simulink model "UAV_SIL"  (R2016b)
settings: Solver=VariableStepAuto  StartTime=0.0  StopTime=10.0  RelTol=1e-3
values from neighbouring files (symbols this model uses):
  MPCSampleTime = 0.02    [matlab.mat]    (also in setup.m)
  TrimCondition =     [matlab.mat]
libraries: Controller_Wrapper x1, Actuator_Lib x1, AircraftModel x1
settings Model: Creator=UAVLAB  LastModifiedBy=UAVLAB

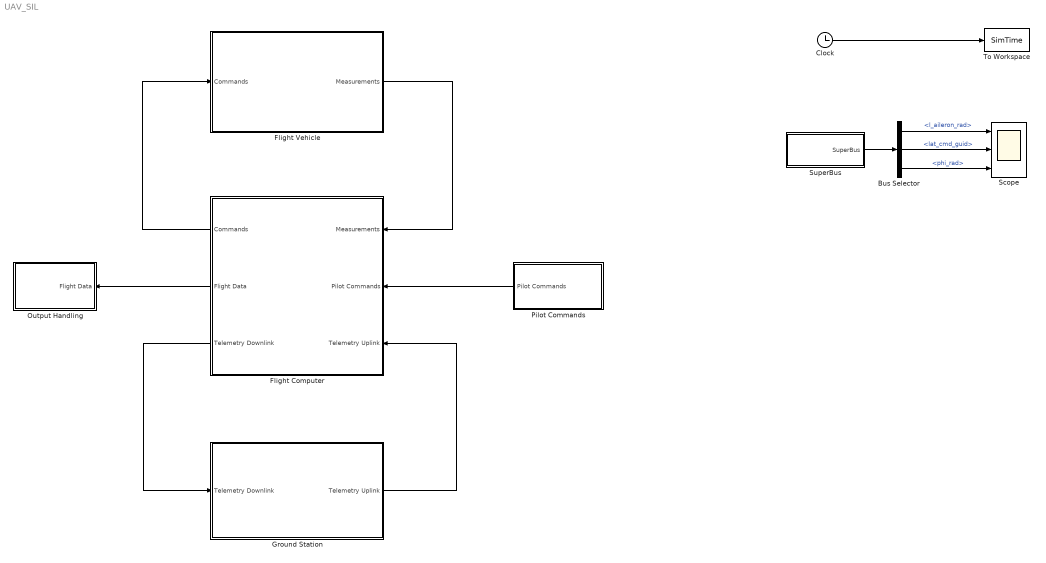
== system UAV_SIL ==
  Bus Selector : BusSelector  OutputSignals=Actuator States.CtrlSurf.l_aileron_rad,References.lat_cmd_guid,Aircraft States.RigidStates.Euler.phi_rad
  Clock : Clock
  Flight Computer : Subsystem
  Flight Vehicle : Subsystem
  Ground Station : Subsystem
  Output Handling : Subsystem
  Pilot Commands : Subsystem
  Scope : Scope  NumInputPorts=3
  SuperBus : Subsystem
  To Workspace : ToWorkspace  VariableName=SimTime  SampleTime=-1
  wires:
  Clock/1 -> To Workspace/1
  SuperBus/1(SuperBus) -> Bus Selector/1
  Flight Vehicle/1(Measurements) -> Flight Computer/1(Measurements)
  Pilot Commands/1(Pilot Commands) -> Flight Computer/2(Pilot Commands)
  Ground Station/1(Telemetry Uplink) -> Flight Computer/3(Telemetry Uplink)
  Flight Computer/1(Commands) -> Flight Vehicle/1(Commands)
  Flight Computer/3(Telemetry Downlink) -> Ground Station/1(Telemetry Downlink)
  Flight Computer/2(Flight Data) -> Output Handling/1(Flight Data)
  Bus Selector/1 -> Scope/1  "<l_aileron_rad>"
  Bus Selector/2 -> Scope/2  "<lat_cmd_guid>"
  Bus Selector/3 -> Scope/3  "<phi_rad>"

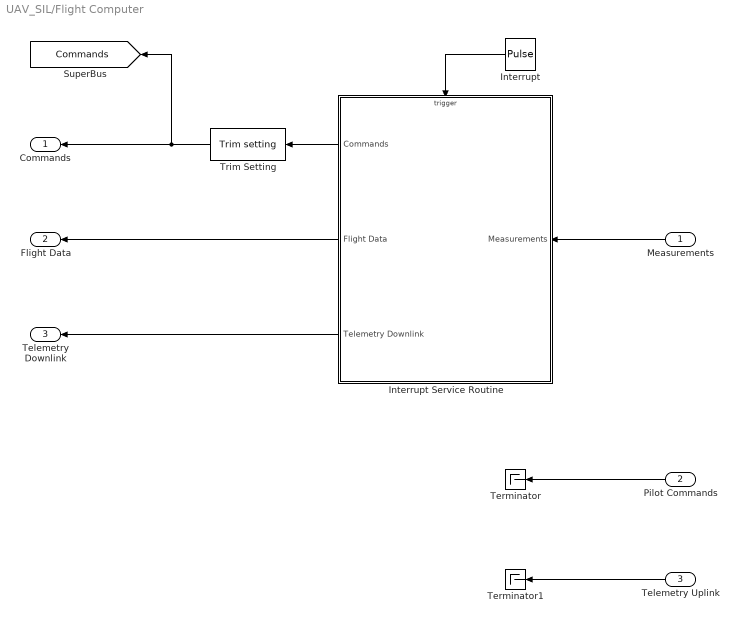
== system UAV_SIL/Flight Computer ==
  Measurements : Inport  OutDataTypeStr=Bus: Sensors
  Pilot Commands : Inport  Port=2  OutDataTypeStr=Bus: PilotCommands
  Telemetry Uplink : Inport  Port=3
  Interrupt : DiscretePulseGenerator  PulseType=Time based  Period=MPCSampleTime  PulseWidth=5
  Interrupt Service Routine : Subsystem  TreatAsAtomicUnit=on
  Terminator : Terminator
  Terminator1 : Terminator
  "Trim Setting " : Actuator_Lib/Trim setting 
  Commands : Outport  OutDataTypeStr=Bus: Commands
  Flight Data : Outport  Port=2
  Telemetry Downlink : Outport  Port=3
  tag scope: Commands=global
  wires:
  Interrupt/1 -> Interrupt Service Routine/Trigger
  Measurements/1 -> Interrupt Service Routine/1(Measurements)
  Interrupt Service Routine/1(Commands) -> "Trim Setting "/1
  "Trim Setting "/1 -> [Commands], Commands/1
  Pilot Commands/1 -> Terminator/1
  Interrupt Service Routine/2(Flight Data) -> Flight Data/1
  Interrupt Service Routine/3(Telemetry Downlink) -> Telemetry Downlink/1
  Telemetry Uplink/1 -> Terminator1/1

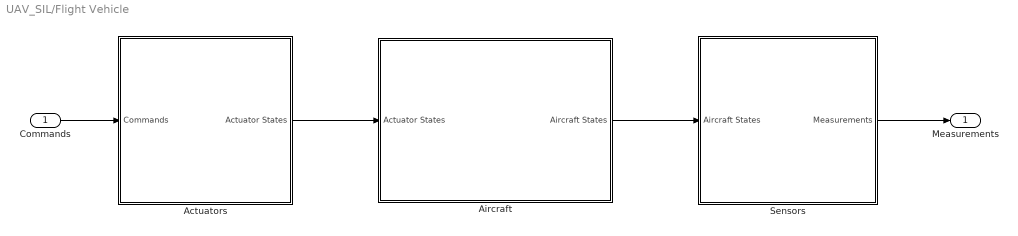
== system UAV_SIL/Flight Vehicle ==
  Commands : Inport  OutDataTypeStr=Bus: Commands
  Actuators : Subsystem
  Aircraft : Subsystem
  Sensors : Subsystem
  Measurements : Outport  OutDataTypeStr=Bus: Sensors  LockScale=on
  wires:
  Sensors/1(Measurements) -> Measurements/1
  Commands/1 -> Actuators/1(Commands)
  Actuators/1(Actuator States) -> Aircraft/1(Actuator States)
  Aircraft/1(Aircraft States) -> Sensors/1(Aircraft States)

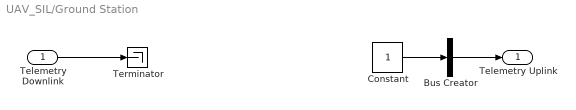
== system UAV_SIL/Ground Station ==
  Telemetry Downlink : Inport
  Bus Creator : BusCreator  Inputs=1
  Constant : Constant
  Terminator : Terminator
  Telemetry Uplink : Outport
  wires:
  Telemetry Downlink/1 -> Terminator/1
  Constant/1 -> Bus Creator/1
  Bus Creator/1 -> Telemetry Uplink/1

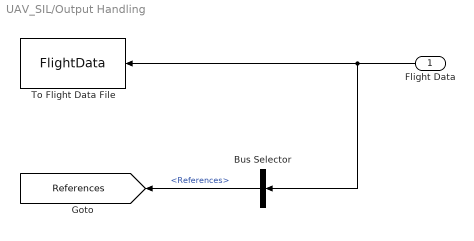
== system UAV_SIL/Output Handling ==
  Flight Data : Inport
  Bus Selector : BusSelector  OutputSignals=References
  To Flight Data File : ToWorkspace  VariableName=FlightData  SaveFormat=Structure With Time  SampleTime=-1
  tag scope: References=global
  wires:
  Flight Data/1 -> Bus Selector/1, To Flight Data File/1
  Bus Selector/1 -> [References]  "<References>"

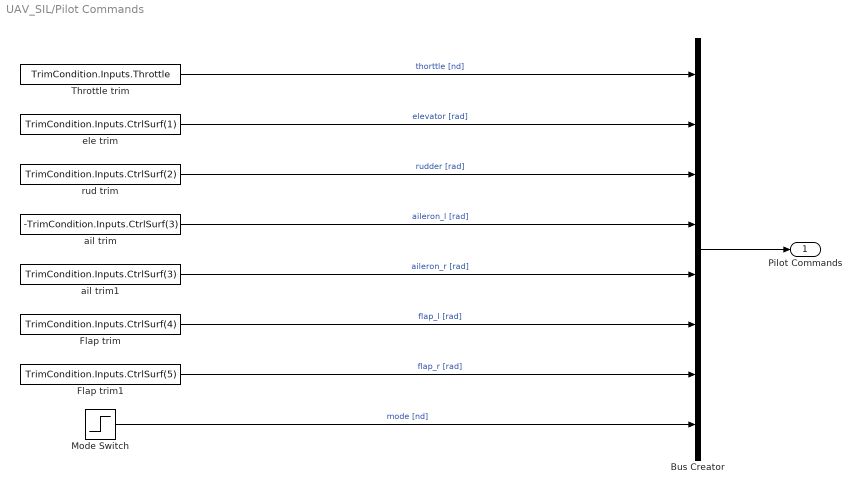
== system UAV_SIL/Pilot Commands ==
  Bus Creator : BusCreator  Inputs=8  OutDataTypeStr=Bus: PilotCommands
      settings: InheritFromInputs=off
  Flap trim : Constant  Value=TrimCondition.Inputs.CtrlSurf(4)
  Flap trim1 : Constant  Value=TrimCondition.Inputs.CtrlSurf(5)  SampleTime=-1
  Mode Switch : Step  Time=3  SampleTime=0
  Throttle trim : Constant  Value=TrimCondition.Inputs.Throttle  SampleTime=-1
  ail trim : Constant  Value=-TrimCondition.Inputs.CtrlSurf(3)  SampleTime=-1
  ail trim1 : Constant  Value=TrimCondition.Inputs.CtrlSurf(3)  SampleTime=-1
  ele trim : Constant  Value=TrimCondition.Inputs.CtrlSurf(1)  SampleTime=-1
  rud trim : Constant  Value=TrimCondition.Inputs.CtrlSurf(2)  SampleTime=-1
  Pilot Commands : Outport  OutDataTypeStr=Bus: PilotCommands
  wires:
  Bus Creator/1 -> Pilot Commands/1
  Flap trim/1 -> Bus Creator/6  "flap_l [rad]"
  ail trim1/1 -> Bus Creator/5  "aileron_r [rad]"
  ail trim/1 -> Bus Creator/4  "aileron_l [rad]"
  rud trim/1 -> Bus Creator/3  "rudder [rad]"
  ele trim/1 -> Bus Creator/2  "elevator [rad]"
  Mode Switch/1 -> Bus Creator/8  "mode [nd]"
  Flap trim1/1 -> Bus Creator/7  "flap_r [rad]"
  Throttle trim/1 -> Bus Creator/1  "thorttle [nd]"

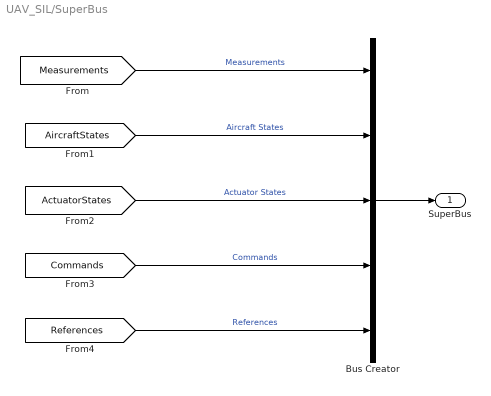
== system UAV_SIL/SuperBus ==
  Bus Creator : BusCreator  Inputs=5
  SuperBus : Outport
  wires:
  [References] -> Bus Creator/5  "References"
  [Commands] -> Bus Creator/4  "Commands"
  [ActuatorStates] -> Bus Creator/3  "Actuator States"
  [AircraftStates] -> Bus Creator/2  "Aircraft States"
  [Measurements] -> Bus Creator/1  "Measurements"
  Bus Creator/1 -> SuperBus/1

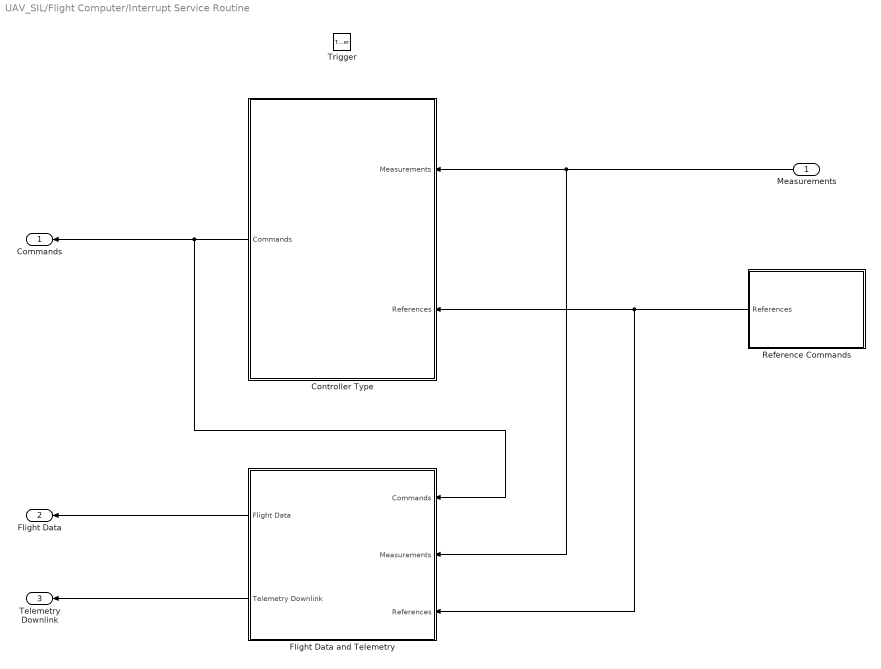
== system UAV_SIL/Flight Computer/Interrupt Service Routine ==
  Measurements : Inport  OutDataTypeStr=Bus: Sensors  LatchByDelayingOutsideSignal=on
  Trigger : TriggerPort  VariantControl=Variant
  Controller Type : Subsystem  BlockChoice=C Code
      settings: AttributesFormatString=%<BlockChoice>  TemplateBlock=Controller_Wrapper/Controller  MemberBlocks=C Code,Simulink
  Flight Data and Telemetry : Subsystem
  Reference Commands : Subsystem
  Commands : Outport  OutDataTypeStr=Bus: Commands
  Flight Data : Outport  Port=2
  Telemetry Downlink : Outport  Port=3
  wires:
  Measurements/1 -> Flight Data and Telemetry/2(Measurements), Controller Type/1(Measurements)
  Reference Commands/1(References) -> Flight Data and Telemetry/3(References), Controller Type/2(References)
  Controller Type/1(Commands) -> Flight Data and Telemetry/1(Commands), Commands/1
  Flight Data and Telemetry/2(Telemetry Downlink) -> Telemetry Downlink/1
  Flight Data and Telemetry/1(Flight Data) -> Flight Data/1

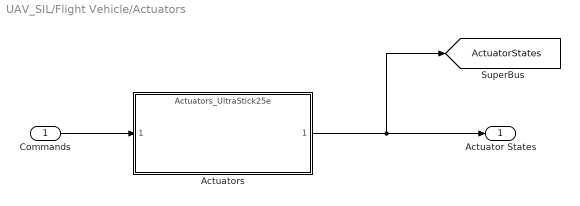
== system UAV_SIL/Flight Vehicle/Actuators ==
  Commands : Inport  OutDataTypeStr=Bus: Commands
  Actuators : ModelReference  ModelNameDialog=Actuators_UltraStick25e  SimulationMode=Normal  Variant=on  ModelReferenceVersion=1.2
  Actuator States : Outport  OutDataTypeStr=Bus: Actuators
  tag scope: ActuatorStates=global
  wires:
  Actuators/1 -> [ActuatorStates], Actuator States/1
  Commands/1 -> Actuators/1

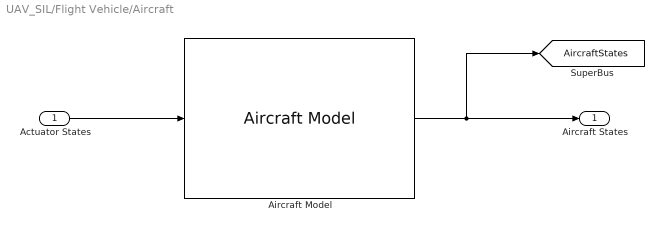
== system UAV_SIL/Flight Vehicle/Aircraft ==
  Actuator States : Inport  OutDataTypeStr=Bus: Actuators
  Aircraft Model : AircraftModel/Aircraft Model
  Aircraft States : Outport  OutDataTypeStr=Bus: States
  tag scope: AircraftStates=global
  wires:
  Actuator States/1 -> Aircraft Model/1
  Aircraft Model/1 -> Aircraft States/1, [AircraftStates]

== system UAV_SIL/Flight Vehicle/Sensors ==
  Aircraft States : Inport  OutDataTypeStr=Bus: States
  Sensor Model : ModelReference  ModelNameDialog=Sensors_UltraStick25e  SimulationMode=Normal  Variant=on  ModelReferenceVersion=1.20
  Measurements : Outport  OutDataTypeStr=Bus: Sensors
  tag scope: Measurements=global
  wires:
  Sensor Model/1 -> [Measurements], Measurements/1
  Aircraft States/1 -> Sensor Model/1

== system UAV_SIL/Flight Computer/Interrupt Service Routine/Controller Type ==
  Measurements : Inport
  References : Inport  Port=2
  C Code : Controller_Wrapper/C Code
  Commands : Outport
  wires:
  Measurements/1 -> C Code/1
  References/1 -> C Code/2
  C Code/1 -> Commands/1

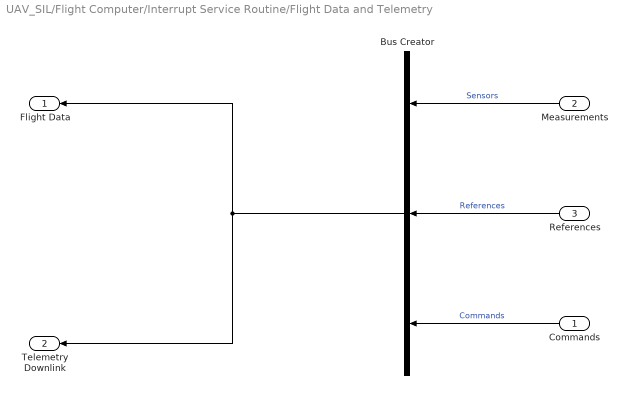
== system UAV_SIL/Flight Computer/Interrupt Service Routine/Flight Data and Telemetry ==
  Commands : Inport  OutDataTypeStr=Bus: Commands
  Measurements : Inport  Port=2  OutDataTypeStr=Bus: Sensors
  References : Inport  Port=3  OutDataTypeStr=Bus: Refs
  Bus Creator : BusCreator  Inputs=3
  Flight Data : Outport
  Telemetry Downlink : Outport  Port=2
  wires:
  Bus Creator/1 -> Flight Data/1, Telemetry Downlink/1
  Measurements/1 -> Bus Creator/1  "Sensors"
  References/1 -> Bus Creator/2  "References"
  Commands/1 -> Bus Creator/3  "Commands"

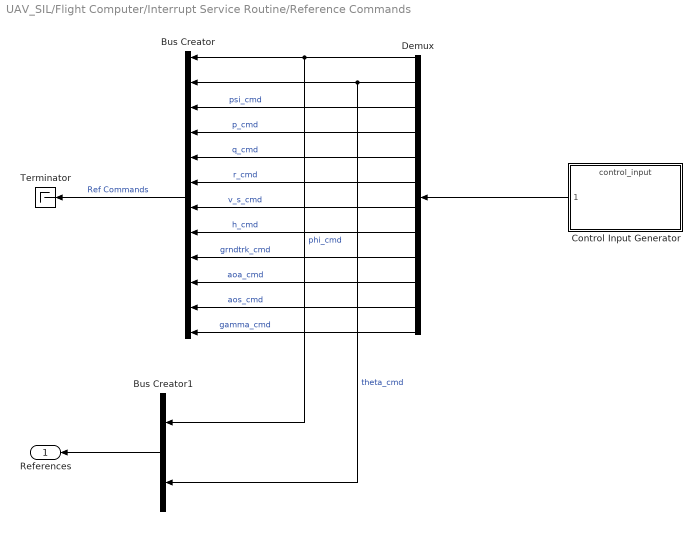
== system UAV_SIL/Flight Computer/Interrupt Service Routine/Reference Commands ==
  Bus Creator : BusCreator  Inputs=12
  Bus Creator1 : BusCreator  Inputs=2  OutDataTypeStr=Bus: Refs
      settings: InheritFromInputs=off
  Control Input Generator : ModelReference  ModelNameDialog=control_input  SimulationMode=Normal  ModelReferenceVersion=1.13
  Demux : Demux  Outputs=12
  Terminator : Terminator
  References : Outport  OutDataTypeStr=Bus: Refs
  wires:
  Control Input Generator/1 -> Demux/1
  Demux/12 -> Bus Creator/12  "gamma_cmd"
  Demux/11 -> Bus Creator/11  "aos_cmd"
  Demux/10 -> Bus Creator/10  "aoa_cmd"
  Demux/9 -> Bus Creator/9  "grndtrk_cmd"
  Demux/8 -> Bus Creator/8  "h_cmd"
  Demux/7 -> Bus Creator/7  "v_s_cmd"
  Demux/6 -> Bus Creator/6  "r_cmd"
  Demux/5 -> Bus Creator/5  "q_cmd"
  Demux/4 -> Bus Creator/4  "p_cmd"
  Demux/3 -> Bus Creator/3  "psi_cmd"
  Demux/2 -> Bus Creator1/2, Bus Creator/2  "theta_cmd"
  Demux/1 -> Bus Creator1/1, Bus Creator/1  "phi_cmd"
  Bus Creator/1 -> Terminator/1  "Ref Commands"
  Bus Creator1/1 -> References/1
